simulink model "reto1"  (R2024a)
settings: Solver=VariableStepAuto  StartTime=0.0  StopTime=10.0  RelTol=1e-3
settings Model: Creator=Usuario  LastModifiedBy=Usuario

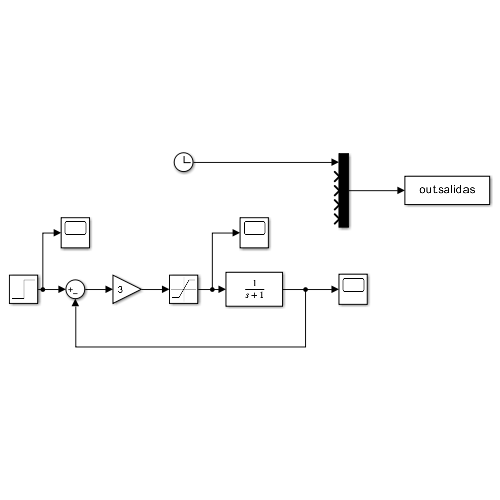
[thumbnail: Simulink's stored preview of the top-level diagram]
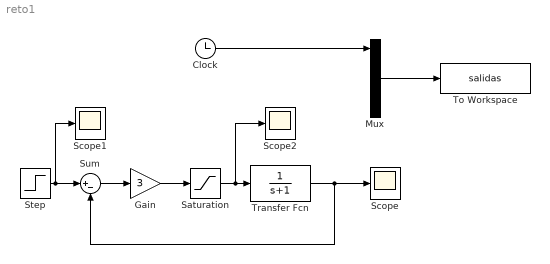
== system reto1 ==
  Clock : Clock
  Gain : Gain  Gain=3
  Mux : Mux  Inputs=5
  Saturation : Saturate  UpperLimit=5  LowerLimit=-5
  Scope : Scope
  Scope1 : Scope
  Scope2 : Scope
  Step : Step  Time=0  SampleTime=0
  Sum : Sum  Inputs=|+-
  To Workspace : ToWorkspace  VariableName=salidas  SampleTime=-1
  Transfer Fcn : TransferFcn  Denominator=[1 1]
  wires:
  Sum/1 -> Gain/1
  Transfer Fcn/1 -> Sum/2, Scope/1
  Step/1 -> Scope1/1, Sum/1
  Clock/1 -> Mux/1
  Mux/1 -> To Workspace/1
  Gain/1 -> Saturation/1
  Saturation/1 -> Scope2/1, Transfer Fcn/1
